simulink library "APST_Lib"  (R2016a)
settings: Solver=ode45  StartTime=0.0  StopTime=10.0  RelTol=1e-3
undefined symbols (not defined in the file or in its folder): ACM, COMP_MAP, rev_comms_sink
libraries: APST_Lib x97
(part 1 of 6)
settings Model: Creator=mwillms4  LastModifiedBy=mwillms4
settings DataIOCC: LimitDataPoints=on
settings DebuggingCC: AllowSymbolicDim=off

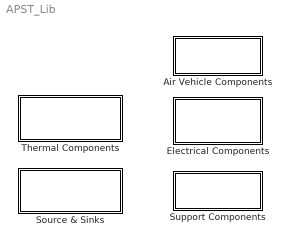
== system APST_Lib ==
  Air Vehicle Components : Subsystem
  Electrical Components : Subsystem
  Source & Sinks : Subsystem
  Support Components : Subsystem
  Thermal Components : Subsystem

== system APST_Lib/Air Vehicle Components ==
  Aircraft : Subsystem  mask(Fluid Tank){Vel_init=300, M_dry=108500, M_load=21337, rho=0.243, A=360, Cd=0.02439}
      mask prompts: Vel_init "Initial Velocity [m/s]"; M_dry "Dry Weight [kg]"; M_load "Payload Weight [kg]"; rho "Air Density [kg/m^3]"; A "Reference Area [m²]"; Cd "Drag Coefficient [-]"
      mask help: Tracks the time rate of change for fluid mass and temperature.
      settings: OpenFcn=|
      | load('Fluids.mat');
      | Set_Fluid_Popup_Names( Fluid )
      mask DialogControl Container8 Prompt: Parameters
      mask Display:
      | image(imread('aircraft.jpg'))
      | 
      | text(0.5,0.9,['{\bf Aircraft}'],'TexMode','on','horizontalAlignment', 'center')
      | 
      | port_label('input',1,'Fuel Mass [kg]')
      | port_label('output',1,'Right Engine')
      | port_label('output',2,'Left Engine')
  Engine : Subsystem  mask(Fluid Tank){fuel=Fuel, P=3500, Omega_init=1000, J=100, Omega_max=1500, Thrust_max=100000, eta=0.25, alpha=0.15}
      mask prompts: fuel "Fuel Type"; P "Engine Pressure [kPa]"; Omega_init "Initial Shaft Speed [rad/s]"; J "Moment of Inertia [kg m²]"; Omega_max "Maximum Shaft Speed [rad/s]"; Thrust_max "Maximum Thrust [N]"; eta "Engine Efficiency [-]"; alpha "Bearing Heat Gen Coeff. [kW/rad/s]"
      mask help: Tracks the time rate of change for fluid mass and temperature.
      mask init:
      | load('Fluids.mat');
      | Fuel = eval(['Fluid.',fuel]);
      settings: OpenFcn=|
      | load('Fluids.mat');
      | Set_Fluid_Popup_Names( Fluid )
      mask TypeOptions fuel: Fuel | Water | Air | PG50
      mask DialogControl Container9 Prompt: Engine Parameters
      mask Display:
      | image(imread('engine.jpg'))
      | 
      | text(0.5,0.9,['{\bf Engine}'],'TexMode','on','horizontalAlignment', 'center')
      | text(0.5,0.1,['{(P)}'],'TexMode','on','horizontalAlignment', 'center')
      | 
      | port_label('input',1,'Aircraft')
      | port_label('input',2,'Fuel In')
      | port_label('output',1,'Generator')
      | port_label('output',2,'Heat')

== system APST_Lib/Electrical Components ==
  Battery : Subsystem  mask{SOC0=0, C=100, P_max=100, T0=20, eta_max=0.98, T_max=100, eta_min=0.8}
      mask prompts: SOC0 "Initial State of Charge [0:1]"; C "Capacitance [MJ]"; P_max "Maximum Power [kW]"; T0 "Maximum Efficiency Temperature [oC]"; eta_max "Maximum Efficiency [0:1]"; T_max "Maximum Temperature [oC]"; eta_min "Minimum Efficiency [0:1]"
      mask init:
      | a = -(eta_max-eta_min)/(T_max-T0)^2;
      | b = -2*a*T0;
      | c = eta_max + a*T0^2;
      mask Display:
      | % text(0.5,0.9,['{\bf Load}'],'TexMode','on','horizontalAlignment', 'center')
      | 
      | port_label('input',1,'Power')
      | port_label('input',2,'Usage')
      | port_label('output',1,'Heat')
  Bus1 : Subsystem  mask(Bus){}
      mask help: This is a bus.
  Converter : Subsystem  mask(Fluid Tank){V=230, I0=100, eta_max=0.98, eta_min=0.8}
      mask prompts: V "Converter Voltage [V]"; I0 "Maximum Efficiency Current [A]"; eta_max "Maximum Efficiency [0:1]"; eta_min "Minimum Efficiency [0:1]"
      mask help: Tracks the time rate of change for fluid mass and temperature.
      settings: OpenFcn=|
      | load('Fluids.mat');
      | Set_Fluid_Popup_Names( Fluid )
      mask DialogControl Container9 Prompt: Converter Parameters
      mask Display:
      | % image(imread('inverter.jpg'))
      | 
      | text(0.5,0.9,['{\bf Inverter}'],'TexMode','on','horizontalAlignment', 'center')
      | 
      | port_label('input',1,'In')
      | port_label('output',1,'Out')
      | port_label('output',2,'Heat')
  Dist : Subsystem
  Generator : Subsystem  mask(Fluid Tank){V=230, eta=0.98}
      mask prompts: V "Generator Voltage"; eta "Generator Efficiency"
      mask help: Tracks the time rate of change for fluid mass and temperature.
      settings: OpenFcn=|
      | load('Fluids.mat');
      | Set_Fluid_Popup_Names( Fluid )
      mask DialogControl Container9 Prompt: Generator Parameters
      mask Display:
      | image(imread('generator.jpg'))
      | 
      | text(0.5,0.9,['{\bf Generator}'],'TexMode','on','horizontalAlignment', 'center')
      | 
      | port_label('input',1,'Engine')
      | port_label('output',1,'Bus')
      | port_label('output',2,'Heat')
  Heater : Subsystem  mask{P_max=100}
      mask prompts: P_max "Maximum Power [kW]"
      mask Display:
      | % text(0.5,0.9,['{\bf Load}'],'TexMode','on','horizontalAlignment', 'center')
      | 
      | port_label('input',1,'Power')
      | port_label('input',2,'Usage')
      | port_label('output',1,'Heat')
  Load : Subsystem  mask{P_max=100}
      mask prompts: P_max "Maximum Power [kW]"
      mask Display:
      | % text(0.5,0.9,['{\bf Load}'],'TexMode','on','horizontalAlignment', 'center')
      | 
      | port_label('input',1,'Power')
      | port_label('input',2,'Usage')
  QLoad : Subsystem  mask{P_max=100, T0=20, eta_max=0.98, T_max=100, eta_min=0.8}
      mask prompts: P_max "Maximum Power [kW]"; T0 "Maximum Efficiency Temperature [oC]"; eta_max "Maximum Efficiency [0:1]"; T_max "Maximum Temperature [oC]"; eta_min "Minimum Efficiency [0:1]"
      mask init:
      | a = -(eta_max-eta_min)/(T_max-T0)^2;
      | b = -2*a*T0;
      | c = eta_max + a*T0^2;
      mask Display:
      | % text(0.5,0.9,['{\bf Load}'],'TexMode','on','horizontalAlignment', 'center')
      | 
      | port_label('input',1,'Power')
      | port_label('input',2,'Usage')
      | port_label('output',1,'Heat')
  Switch : Subsystem  mask(Switch){}
      mask help: This is a switch.

== system APST_Lib/Source & Sinks ==
  Flow Flow Source (Pressure) : Subsystem  mask(Flow Source (Pressure)){M_ext=on, M=0, T_ext=on, T=0, P_ext=on, P=0}
      mask prompts: M_ext "Mass flow rate time varying?"; M "Mass flow rate (kg/s)"; T_ext "Temperature time varying?"; T "Temperature (C)"; P_ext "Pressure time varying?"; P "Pressure (kPa)"
      mask help: Used to create a flow source.
      mask Callback M_ext:
      | en = get_param(gcb,'MaskVisibilities');
      | h      = get_param(gcb,'handle');   % Get block handle
      | blk    = gcb;
      | hblock = get(h);     % Parse out handles structure
      | 
      | switch get_param(gcb,'M_ext')
      |     case 'on'
      |         en{2} = 'off';
      |         %add_block('simulink/Ports & Subsystems/In1',   [blk,'/In1'],'Position',[130    -7   160     7]);         % adding inport
      | 
      |     case 'off'
      |         en{2} = 'on';
      |         %delete_block([blk,'/In1'])
      | 
      | end
      | set_param(gcb,'MaskVisibilities',en);
      mask Callback T_ext:
      | en = get_param(gcb,'MaskVisibilities');
      | 
      | switch get_param(gcb,'T_ext')
      |     case 'on'
      |         en{4} = 'off';
      |     case 'off'
      |         en{4} = 'on';
      | end
      | set_param(gcb,'MaskVisibilities',en);
      mask Callback P_ext:
      | en = get_param(gcb,'MaskVisibilities');
      | 
      | switch get_param(gcb,'P_ext')
      |     case 'on'
      |         en{6} = 'off';
      |     case 'off'
      |         en{6} = 'on';
      | end
      | set_param(gcb,'MaskVisibilities',en);
      mask Display:
      | text(0.5,0.95,['{\bf Pressure Source}'],'TexMode','on','horizontalAlignment', 'center')
      | text(0.5,0.1,['{(start)}'],'TexMode','on','horizontalAlignment', 'center')
      | 
      | port_label('input',1,'Source Temperature (C)')
      | port_label('input',2,'Source Pressure (kPa)')
      | 
      | port_label('output',1,'Source')
  Flow Sink (Generic) : Subsystem  mask(Flow Sink (Mass Flow Rate)){M_ext=on, M=0, T_ext=on, T=0, P_ext=on, P=0}
      mask prompts: M_ext "Mass flow rate time varying?"; M "Mass flow rate (kg/s)"; T_ext "Temperature time varying?"; T "Temperature (C)"; P_ext "Pressure time varying?"; P "Pressure (kPa)"
      mask help: Used to create a flow sink.
      mask Callback M_ext:
      | en = get_param(gcb,'MaskVisibilities');
      | h      = get_param(gcb,'handle');   % Get block handle
      | blk    = gcb;
      | hblock = get(h);     % Parse out handles structure
      | 
      | switch get_param(gcb,'M_ext')
      |     case 'on'
      |         en{2} = 'off';
      |         %add_block('simulink/Ports & Subsystems/In1',   [blk,'/In1'],'Position',[130    -7   160     7]);         % adding inport
      | 
      |     case 'off'
      |         en{2} = 'on';
      |         %delete_block([blk,'/In1'])
      | 
      | end
      | set_param(gcb,'MaskVisibilities',en);
      mask Callback T_ext:
      | en = get_param(gcb,'MaskVisibilities');
      | 
      | switch get_param(gcb,'T_ext')
      |     case 'on'
      |         en{4} = 'off';
      |     case 'off'
      |         en{4} = 'on';
      | end
      | set_param(gcb,'MaskVisibilities',en);
      mask Callback P_ext:
      | en = get_param(gcb,'MaskVisibilities');
      | 
      | switch get_param(gcb,'P_ext')
      |     case 'on'
      |         en{6} = 'off';
      |     case 'off'
      |         en{6} = 'on';
      | end
      | set_param(gcb,'MaskVisibilities',en);
      mask Display:
      | text(0.5,0.95,['{\bf Generic Sink}'],'TexMode','on','horizontalAlignment', 'center')
      | text(0.5,0.1,['{-----end}'],'TexMode','on','horizontalAlignment', 'center')
      | 
      | port_label('input',1,'Sink')
      | port_label('input',2,'Sink Value')
  Flow Sink (Mass Flow Rate) : Subsystem  mask(Flow Sink (Mass Flow Rate)){M_ext=on, M=0, T_ext=on, T=0, P_ext=on, P=0}
      mask prompts: M_ext "Mass flow rate time varying?"; M "Mass flow rate (kg/s)"; T_ext "Temperature time varying?"; T "Temperature (C)"; P_ext "Pressure time varying?"; P "Pressure (kPa)"
      mask help: Used to create a flow sink.
      mask Callback M_ext:
      | en = get_param(gcb,'MaskVisibilities');
      | h      = get_param(gcb,'handle');   % Get block handle
      | blk    = gcb;
      | hblock = get(h);     % Parse out handles structure
      | 
      | switch get_param(gcb,'M_ext')
      |     case 'on'
      |         en{2} = 'off';
      |         %add_block('simulink/Ports & Subsystems/In1',   [blk,'/In1'],'Position',[130    -7   160     7]);         % adding inport
      | 
      |     case 'off'
      |         en{2} = 'on';
      |         %delete_block([blk,'/In1'])
      | 
      | end
      | set_param(gcb,'MaskVisibilities',en);
      mask Callback T_ext:
      | en = get_param(gcb,'MaskVisibilities');
      | 
      | switch get_param(gcb,'T_ext')
      |     case 'on'
      |         en{4} = 'off';
      |     case 'off'
      |         en{4} = 'on';
      | end
      | set_param(gcb,'MaskVisibilities',en);
      mask Callback P_ext:
      | en = get_param(gcb,'MaskVisibilities');
      | 
      | switch get_param(gcb,'P_ext')
      |     case 'on'
      |         en{6} = 'off';
      |     case 'off'
      |         en{6} = 'on';
      | end
      | set_param(gcb,'MaskVisibilities',en);
      mask Display:
      | text(0.5,0.95,['{\bf Mass Flow Rate Sink}'],'TexMode','on','horizontalAlignment', 'center')
      | text(0.5,0.1,['{-----end}'],'TexMode','on','horizontalAlignment', 'center')
      | 
      | port_label('input',1,'Sink')
      | port_label('input',2,'Sink Mass Flow Rate (kg/s)')
  Flow Sink (Pressure) : Subsystem  mask(Flow Sink (Pressure)){M_ext=on, M=0, T_ext=on, T=0, P_ext=on, P=0}
      mask prompts: M_ext "Mass flow rate time varying?"; M "Mass flow rate (kg/s)"; T_ext "Temperature time varying?"; T "Temperature (C)"; P_ext "Pressure time varying?"; P "Pressure (kPa)"
      mask help: Used to create a flow sink.
      mask Callback M_ext:
      | en = get_param(gcb,'MaskVisibilities');
      | h      = get_param(gcb,'handle');   % Get block handle
      | blk    = gcb;
      | hblock = get(h);     % Parse out handles structure
      | 
      | switch get_param(gcb,'M_ext')
      |     case 'on'
      |         en{2} = 'off';
      |         %add_block('simulink/Ports & Subsystems/In1',   [blk,'/In1'],'Position',[130    -7   160     7]);         % adding inport
      | 
      |     case 'off'
      |         en{2} = 'on';
      |         %delete_block([blk,'/In1'])
      | 
      | end
      | set_param(gcb,'MaskVisibilities',en);
      mask Callback T_ext:
      | en = get_param(gcb,'MaskVisibilities');
      | 
      | switch get_param(gcb,'T_ext')
      |     case 'on'
      |         en{4} = 'off';
      |     case 'off'
      |         en{4} = 'on';
      | end
      | set_param(gcb,'MaskVisibilities',en);
      mask Callback P_ext:
      | en = get_param(gcb,'MaskVisibilities');
      | 
      | switch get_param(gcb,'P_ext')
      |     case 'on'
      |         en{6} = 'off';
      |     case 'off'
      |         en{6} = 'on';
      | end
      | set_param(gcb,'MaskVisibilities',en);
      mask Display:
      | text(0.5,0.95,['{\bf Pressure Sink}'],'TexMode','on','horizontalAlignment', 'center')
      | text(0.5,0.1,['{(end)}'],'TexMode','on','horizontalAlignment', 'center')
      | 
      | port_label('input',1,'Sink')
      | port_label('input',2,'Sink Pressure (kPa)')
  Flow Source (Mass Flow Rate) : Subsystem  mask(Flow Source (Mass Flow Rate)){M_ext=on, M=0, T_ext=on, T=0, P_ext=on, P=0}
      mask prompts: M_ext "Mass flow rate time varying?"; M "Mass flow rate (kg/s)"; T_ext "Temperature time varying?"; T "Temperature (C)"; P_ext "Pressure time varying?"; P "Pressure (kPa)"
      mask help: Used to create a flow source.
      mask Callback M_ext:
      | en = get_param(gcb,'MaskVisibilities');
      | h      = get_param(gcb,'handle');   % Get block handle
      | blk    = gcb;
      | hblock = get(h);     % Parse out handles structure
      | 
      | switch get_param(gcb,'M_ext')
      |     case 'on'
      |         en{2} = 'off';
      |         %add_block('simulink/Ports & Subsystems/In1',   [blk,'/In1'],'Position',[130    -7   160     7]);         % adding inport
      | 
      |     case 'off'
      |         en{2} = 'on';
      |         %delete_block([blk,'/In1'])
      | 
      | end
      | set_param(gcb,'MaskVisibilities',en);
      mask Callback T_ext:
      | en = get_param(gcb,'MaskVisibilities');
      | 
      | switch get_param(gcb,'T_ext')
      |     case 'on'
      |         en{4} = 'off';
      |     case 'off'
      |         en{4} = 'on';
      | end
      | set_param(gcb,'MaskVisibilities',en);
      mask Callback P_ext:
      | en = get_param(gcb,'MaskVisibilities');
      | 
      | switch get_param(gcb,'P_ext')
      |     case 'on'
      |         en{6} = 'off';
      |     case 'off'
      |         en{6} = 'on';
      | end
      | set_param(gcb,'MaskVisibilities',en);
      mask Display:
      | text(0.5,0.95,['{\bf Mass Flow Rate Source}'],'TexMode','on','horizontalAlignment', 'center')
      | text(0.5,0.1,['{start-----}'],'TexMode','on','horizontalAlignment', 'center')
      | 
      | port_label('input',1,'Source Temperature (C)')
      | port_label('input',2,'Source Mass Flow Rate (kg/s)')
      | 
      | port_label('output',1,'Source')
